simulink model "double_integrator_pd"  (R2020b)
settings: Solver=VariableStepAuto  StartTime=0.0  StopTime=10.0  RelTol=1e-3
libraries: simulink x1
settings Model: Creator=nijil  LastModifiedBy=nijil

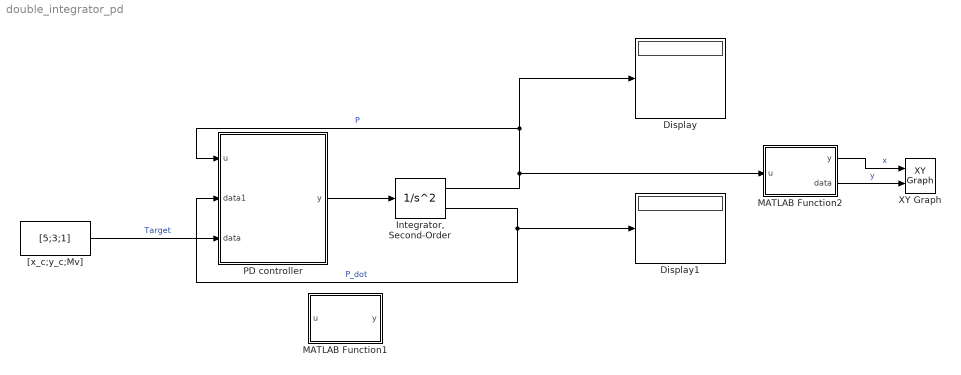
== system double_integrator_pd ==
  Display : Display
  Display1 : Display
  "Integrator, Second-Order" : SecondOrderIntegrator
  MATLAB Function1 : MATLAB Function  TreatAsAtomicUnit=on
  MATLAB Function2 : MATLAB Function  TreatAsAtomicUnit=on
  PD controller : MATLAB Function  TreatAsAtomicUnit=on
  XY Graph : simulink/Sinks/XY Graph  xmin=-10  xmax=10  ymin=-10  ymax=10  st=-1
  "[x_c;y_c;Mv]" : Constant  Value=[5;3;1]
  wires:
  PD controller/1(y) -> "Integrator, Second-Order"/1
  "[x_c;y_c;Mv]"/1 -> PD controller/3(data)  "Target"
  "Integrator, Second-Order"/1 -> MATLAB Function2/1(u), PD controller/1(u), Display/1  "P"
  "Integrator, Second-Order"/2 -> Display1/1, PD controller/2(data1)  "P_dot"
  MATLAB Function2/1(y) -> XY Graph/1  "x"
  MATLAB Function2/2(data) -> XY Graph/2  "y"

== matlab function double_integrator_pd/PD controller ==
  data: u input; data1 input; y output; data input
function y = fcn(u, data1, data)
%data=[x_c;y_c;M_v] u=[x;y] data1=[x_dot;y_dot]
k1=3;
k2=2;
Cv=data(1:2);
y = -k1*data(3)*(u-Cv)-k2*data1;

== matlab function double_integrator_pd/MATLAB Function2 ==
  data: u input; y output; data output
function [y,data] = fcn(u)
y=u(1);
data = u(2);

== matlab function double_integrator_pd/MATLAB Function1 ==
  data: u input; y output
function y = fcn(u)

y = u;
